simulink model "untitled"  (R2018a)
settings: Solver=ode5  StartTime=0.0  StopTime=100  FixedStep=0.01  RelTol=1e-3
settings Model: Creator=Hungs  LastModifiedBy=Hungs

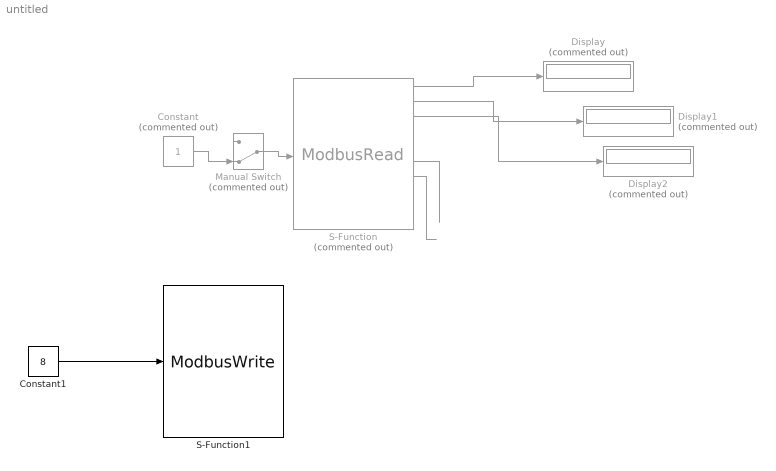
== system untitled ==
  Constant : Constant  Commented=on
  Constant1 : Constant  Value=8
  Display : Display  Commented=on
  Display1 : Display  Commented=on
  Display2 : Display  Commented=on
  Manual Switch : ManualSwitch  Commented=on  CurrentSetting=0
  S-Function : S-Function  Commented=on  FunctionName=ModbusRead  Parameters='127.0.0.1' 502  SFunctionDeploymentMode=off  EnableBusSupport=off
  S-Function1 : S-Function  FunctionName=ModbusWrite  Parameters='127.0.0.1' 502  SFunctionDeploymentMode=off  EnableBusSupport=off
  wires:
  S-Function/6 -> ?
  S-Function/7 -> ?
  S-Function/1 -> Display/1
  S-Function/2 -> Display1/1
  S-Function/3 -> Display2/1
  Manual Switch/1 -> S-Function/1
  Constant/1 -> Manual Switch/2
  Constant1/1 -> S-Function1/1
